simulink model "FIR_Cascade_7"  (R2020b)
settings: Solver=VariableStepAuto  StartTime=0.0  StopTime=10.0  RelTol=1e-3
settings Model: Creator=DELL  LastModifiedBy=DELL

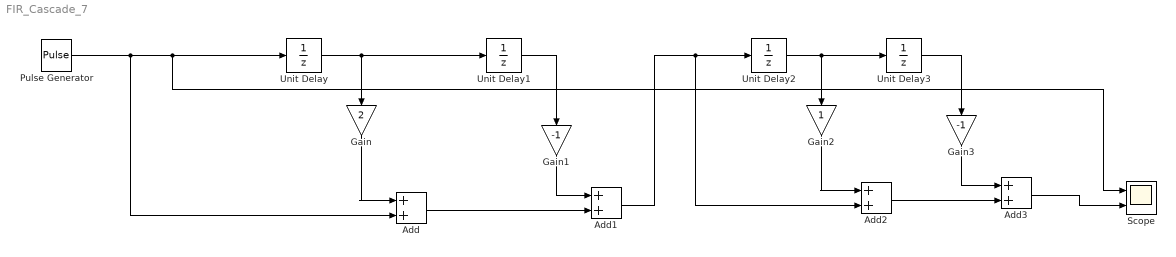
== system FIR_Cascade_7 ==
  Add{,1..3} (4 alike) : Sum
  Gain : Gain  Gain=2
  Gain1 : Gain  Gain=-1
  Gain2 : Gain
  Gain3 : Gain  Gain=-1
  Pulse Generator : DiscretePulseGenerator  PulseType=Time based  Period=1  PulseWidth=20
  Scope : Scope  NumInputPorts=2
  Unit Delay{,1..3} (4 alike) : UnitDelay  SampleTime=-1  HasFrameUpgradeWarning=on
  wires:
  Pulse Generator/1 -> Add/2, Scope/1, Unit Delay/1
  Unit Delay/1 -> Gain/1, Unit Delay1/1
  Add/1 -> Add1/2
  Unit Delay1/1 -> Gain1/1
  Add1/1 -> Add2/2, Unit Delay2/1
  Unit Delay2/1 -> Gain2/1, Unit Delay3/1
  Add2/1 -> Add3/2
  Unit Delay3/1 -> Gain3/1
  Add3/1 -> Scope/2
  Gain/1 -> Add/1
  Gain1/1 -> Add1/1
  Gain2/1 -> Add2/1
  Gain3/1 -> Add3/1
